simulink model "lqg"  (R2024a)
settings: Solver=VariableStepAuto  StartTime=0.0  StopTime=10.0  RelTol=1e-6
values from neighbouring files (symbols this model uses):
  A = [4, -2, 0, 6; -2, 4, -6, 0; 0, -6, 4, 2; 6, 0, 2, 4]    [main.m]
  B = [11, 0; -1, 0; 7, 0; 9, 0]    [main.m]
  C = [1, -1, 1, 1; 1, 3, -1, 3]    [main.m]
  D = [0, 3; 0, 4]    [main.m]
  f = @(t) [3*sin(2*t); 2*cos(3*t); sin(3*t); cos(1*t)]    [main.m]
  K = -R \ B' * P    [TAU.m]
  L = -P * C' / R    [TAU.m]    (also in main.m = TAU.FindObserverKalman(A, C, QL, RL))
  x0 = [1; 1; 1; 1]    [main.m]
settings Model: Creator=alexivanov  LastModifiedBy=alexivanov

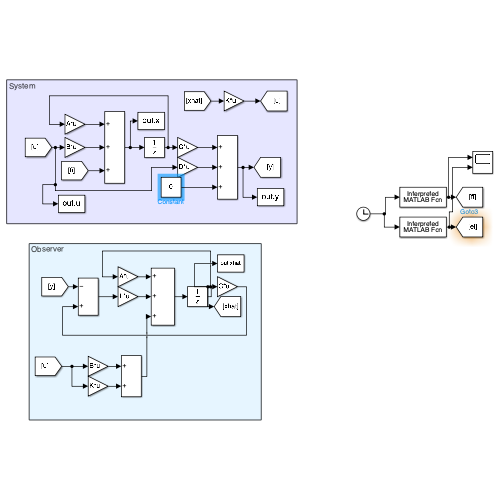
[thumbnail: Simulink's stored preview of the top-level diagram]
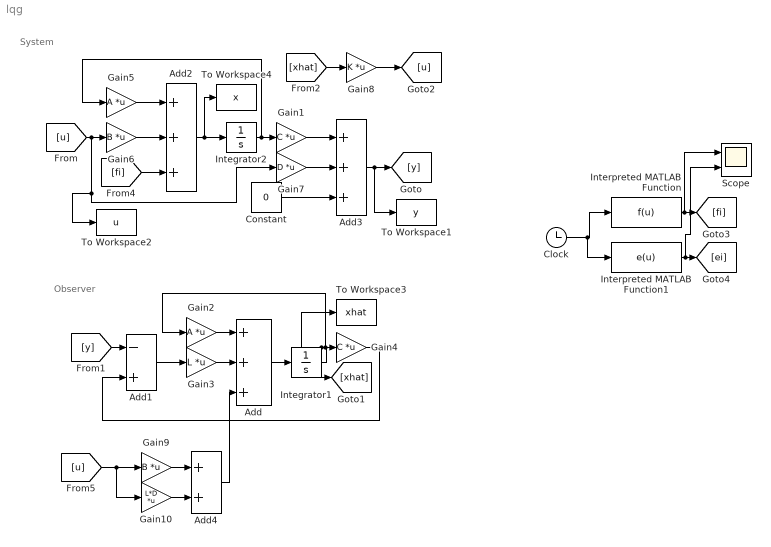
== system lqg ==
  note: System
  note: Observer
  Add : Sum  Inputs=+++
  Add1 : Sum  Inputs=-+
  Add2 : Sum  Inputs=+++
  Add3 : Sum  Inputs=+++
  Add4 : Sum
  Clock : Clock
  Constant : Constant  Value=0
  Gain1 : Gain  Gain=C  Multiplication=Matrix(K*u)
  Gain10 : Gain  Gain=L*D  Multiplication=Matrix(K*u)
  Gain2 : Gain  Gain=A  Multiplication=Matrix(K*u)
  Gain3 : Gain  Gain=L  Multiplication=Matrix(K*u)
  Gain4 : Gain  Gain=C  Multiplication=Matrix(K*u)
  Gain5 : Gain  Gain=A  Multiplication=Matrix(K*u)
  Gain6 : Gain  Gain=B  Multiplication=Matrix(K*u)
  Gain7 : Gain  Gain=D  Multiplication=Matrix(K*u)
  Gain8 : Gain  Gain=K  Multiplication=Matrix(K*u)
  Gain9 : Gain  Gain=B  Multiplication=Matrix(K*u)
  Integrator1 : Integrator
  Integrator2 : Integrator  InitialCondition=x0
  Interpreted MATLAB Function : MATLABFcn  MATLABFcn=f(u)
  Interpreted MATLAB Function1 : MATLABFcn  MATLABFcn=e(u)
  Scope : Scope  NumInputPorts=2
  To Workspace1 : ToWorkspace  VariableName=y  SampleTime=-1
  To Workspace2 : ToWorkspace  VariableName=u  SampleTime=-1
  To Workspace3 : ToWorkspace  VariableName=xhat  SampleTime=-1
  To Workspace4 : ToWorkspace  VariableName=x  SampleTime=-1
  wires:
  Gain4/1 -> Add1/2
  [y] -> Add1/1
  Add/1 -> Integrator1/1
  Integrator1/1 -> [xhat], To Workspace3/1, Gain4/1, Gain2/1
  Add1/1 -> Gain3/1
  Gain2/1 -> Add/1
  Gain3/1 -> Add/2
  Integrator2/1 -> Gain5/1, Gain1/1
  Gain5/1 -> Add2/1
  Gain6/1 -> Add2/2
  [fi] -> Add2/3
  [u] -> To Workspace2/1, Gain7/1, Gain6/1
  Add2/1 -> To Workspace4/1, Integrator2/1
  Gain7/1 -> Add3/2
  Gain1/1 -> Add3/1
  Constant/1 -> Add3/3
  Add3/1 -> To Workspace1/1, [y]
  Gain8/1 -> [u]
  Clock/1 -> Interpreted MATLAB Function1/1, Interpreted MATLAB Function/1
  Interpreted MATLAB Function/1 -> Scope/1, [fi]
  Interpreted MATLAB Function1/1 -> Scope/2, [ei]
  [xhat] -> Gain8/1
  Gain9/1 -> Add4/1
  Gain10/1 -> Add4/2
  [u] -> Gain10/1, Gain9/1
  Add4/1 -> Add/3
